simulink model "CrazyClover_attitude_control_descrete"  (R2020b)
settings: Solver=FixedStepDiscrete  StartTime=0.0  StopTime=1  FixedStep=0.01  RelTol=1e-3
values from neighbouring files (symbols this model uses):
  controller_matrix = [mass/(4*gravity)*1000 mass/(4*gravity)*1000 mass/(4*gravity)*1000 mass/(4*gravity)*1000 ... (first row only)    [sim_param.m]
  kM1 = Armlength /sqrt(2)    [sim_param.m]
  kM2 = Armlength /sqrt(2)    [sim_param.m]
  kM3 = 1    [sim_param.m]
undefined symbols (not defined in the file or in its folder): DiscIntNeverNeededParam, Pitch, Pitchrate, Roll, Rollrate, Yaw, Yawrate
libraries: pid_lib x18
(part 1 of 2)
settings Model: Creator=kt012  LastModifiedBy=kt012

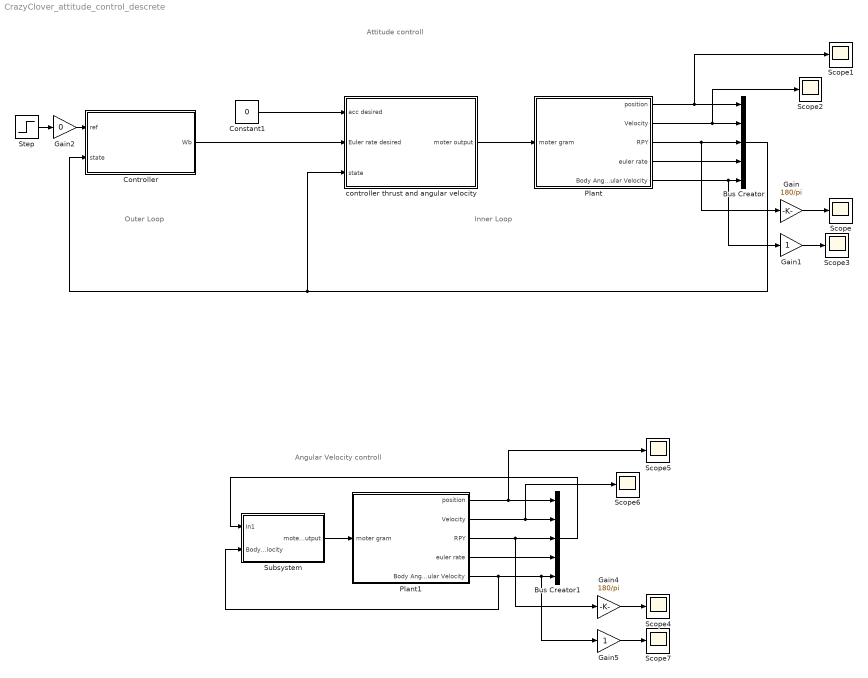
== system CrazyClover_attitude_control_descrete ==
  note: Inner Loop
  note: Outer Loop
  note: Attitude controll
  note: Angular Velocity controll
  Bus Creator : BusCreator  Inputs=5
  Bus Creator1 : BusCreator  Inputs=5
  Constant1 : Constant  Value=0
  Controller : Subsystem
  Gain : Gain  Gain=180/pi
  Gain1 : Gain
  Gain2 : Gain  Gain=0
  Gain4 : Gain  Gain=180/pi
  Gain5 : Gain
  Plant : Subsystem
  Plant1 : Subsystem
  Scope{,1..7} (8 alike) : Scope
  Step : Step  Time=5  Before=[0 0 0]'  After=[1 0 0]'  SampleTime=0
  Subsystem : Subsystem
  controller thrust and angular velocity : Subsystem
  wires:
  Controller/1(Wb) -> controller thrust and angular velocity/2(Euler rate desired)
  Constant1/1 -> controller thrust and angular velocity/1(acc desired)
  Step/1 -> Gain2/1
  Plant/4(euler rate) -> Bus Creator/4
  Plant/2(Velocity) -> Bus Creator/2, Scope2/1
  Plant/3(RPY) -> Gain/1, Bus Creator/3
  Plant/1(position) -> Bus Creator/1, Scope1/1
  controller thrust and angular velocity/1(moter output) -> Plant/1(moter gram)
  Bus Creator/1 -> controller thrust and angular velocity/3(state), Controller/2(state)
  Plant/5(Body Angular Velocity) -> Gain1/1, Bus Creator/5
  Gain/1 -> Scope/1
  Gain1/1 -> Scope3/1
  Gain2/1 -> Controller/1(ref)
  Gain4/1 -> Scope4/1
  Plant1/3(RPY) -> Gain4/1, Bus Creator1/3
  Plant1/5(Body Angular Velocity) -> Subsystem/2(Body Angular Velocity), Gain5/1, Bus Creator1/5
  Plant1/2(Velocity) -> Bus Creator1/2, Scope6/1
  Bus Creator1/1 -> Subsystem/1(In1)
  Plant1/1(position) -> Bus Creator1/1, Scope5/1
  Gain5/1 -> Scope7/1
  Plant1/4(euler rate) -> Bus Creator1/4
  Subsystem/1(moter output) -> Plant1/1(moter gram)

== system CrazyClover_attitude_control_descrete/Controller ==
  ref : Inport
  state : Inport  Port=2
  Subsystem3 : Subsystem
  Wb : Outport
  wires:
  ref/1 -> Subsystem3/1(RPY ref)
  Subsystem3/1(Wb) -> Wb/1
  state/1 -> Subsystem3/2(state)

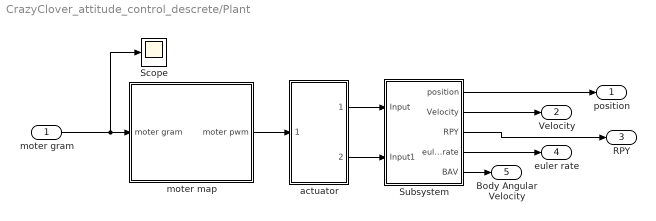
== system CrazyClover_attitude_control_descrete/Plant ==
  moter gram : Inport
  Scope : Scope
  Subsystem : Subsystem
  actuator : Subsystem
  moter map : Subsystem
  position : Outport
  Velocity : Outport  Port=2
  RPY : Outport  Port=3
  euler rate : Outport  Port=4
  Body Angular Velocity : Outport  Port=5
  wires:
  Subsystem/5(BAV) -> Body Angular Velocity/1
  Subsystem/1(position) -> position/1
  Subsystem/3(RPY) -> RPY/1
  moter gram/1 -> Scope/1, moter map/1(moter gram)
  actuator/2(Input1) -> Subsystem/2(Input1)
  actuator/1(Input) -> Subsystem/1(Input)
  moter map/1(moter pwm) -> actuator/1(PWM)
  Subsystem/4(euler rate) -> euler rate/1
  Subsystem/2(Velocity) -> Velocity/1

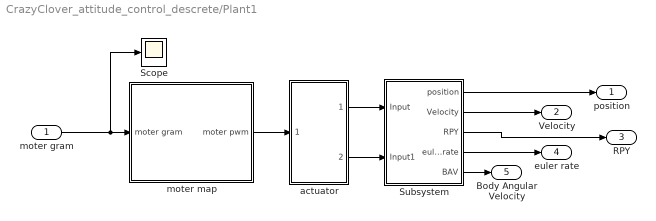
== system CrazyClover_attitude_control_descrete/Plant1 ==
  moter gram : Inport
  Scope : Scope
  Subsystem : Subsystem
  actuator : Subsystem
  moter map : Subsystem
  position : Outport
  Velocity : Outport  Port=2
  RPY : Outport  Port=3
  euler rate : Outport  Port=4
  Body Angular Velocity : Outport  Port=5
  wires:
  moter gram/1 -> Scope/1, moter map/1(moter gram)
  actuator/2(Input1) -> Subsystem/2(Input1)
  Subsystem/4(euler rate) -> euler rate/1
  moter map/1(moter pwm) -> actuator/1(PWM)
  Subsystem/2(Velocity) -> Velocity/1
  Subsystem/3(RPY) -> RPY/1
  Subsystem/1(position) -> position/1
  actuator/1(Input) -> Subsystem/1(Input)
  Subsystem/5(BAV) -> Body Angular Velocity/1

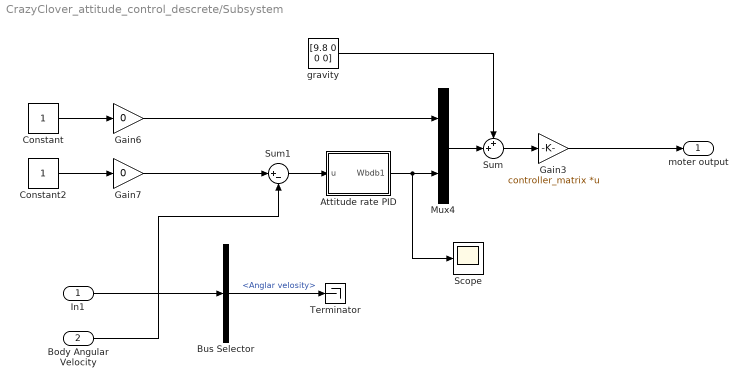
== system CrazyClover_attitude_control_descrete/Subsystem ==
  In1 : Inport
  Body Angular Velocity : Inport  Port=2
  Attitude rate PID : Subsystem
  Bus Selector : BusSelector  OutputSignals=Anglar velosity
  Constant : Constant
  Constant2 : Constant
  Gain3 : Gain  Gain=controller_matrix  Multiplication=Matrix(K*u)
  Gain6 : Gain  Gain=0
  Gain7 : Gain  Gain=0
  Mux4 : Mux  Inputs=2
  Scope : Scope
  Sum : Sum  Inputs=++|
  Sum1 : Sum  Inputs=|+-
  Terminator : Terminator
  gravity : Constant  Value=[9.8 0 0 0]
  moter output : Outport
  wires:
  Attitude rate PID/1(Wbdb1) -> Scope/1, Mux4/2
  Sum/1 -> Gain3/1
  Gain6/1 -> Mux4/1
  Mux4/1 -> Sum/2
  gravity/1 -> Sum/1
  Sum1/1 -> Attitude rate PID/1(u)
  Gain3/1 -> moter output/1
  Constant/1 -> Gain6/1
  Constant2/1 -> Gain7/1
  Gain7/1 -> Sum1/1
  In1/1 -> Bus Selector/1
  Bus Selector/1 -> Terminator/1  "<Anglar velosity>"
  Body Angular Velocity/1 -> Sum1/2

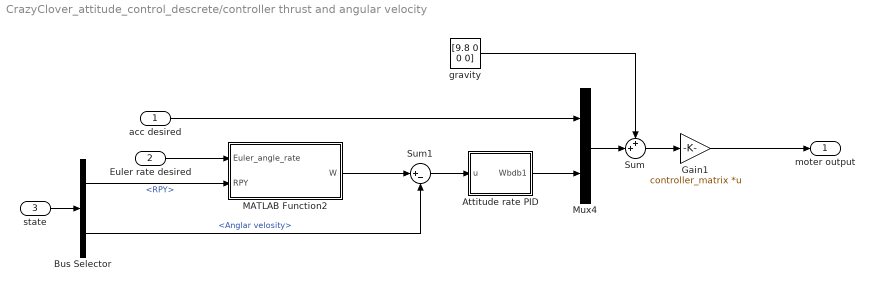
== system CrazyClover_attitude_control_descrete/controller thrust and angular velocity ==
  acc desired : Inport
  Euler rate desired : Inport  Port=2
  state : Inport  Port=3
  Attitude rate PID : Subsystem
  Bus Selector : BusSelector  OutputSignals=RPY,Anglar velosity
  Gain1 : Gain  Gain=controller_matrix  Multiplication=Matrix(K*u)
  MATLAB Function2 : MATLAB Function  TreatAsAtomicUnit=on
  Mux4 : Mux  Inputs=2
  Sum : Sum  Inputs=++|
  Sum1 : Sum  Inputs=|+-
  gravity : Constant  Value=[9.8 0 0 0]
  moter output : Outport
  wires:
  Sum/1 -> Gain1/1
  Gain1/1 -> moter output/1
  Mux4/1 -> Sum/2
  gravity/1 -> Sum/1
  Attitude rate PID/1(Wbdb1) -> Mux4/2
  state/1 -> Bus Selector/1
  Bus Selector/2 -> Sum1/2  "<Anglar velosity>"
  Sum1/1 -> Attitude rate PID/1(u)
  Euler rate desired/1 -> MATLAB Function2/1(Euler_angle_rate)
  acc desired/1 -> Mux4/1
  Bus Selector/1 -> MATLAB Function2/2(RPY)  "<RPY>"
  MATLAB Function2/1(W) -> Sum1/1

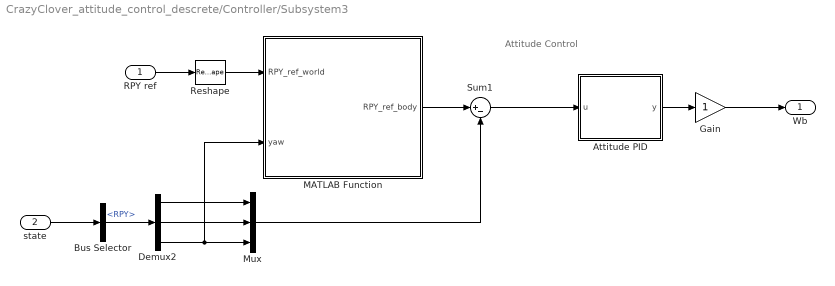
== system CrazyClover_attitude_control_descrete/Controller/Subsystem3 ==
  note: Attitude Control
  RPY ref : Inport
  state : Inport  Port=2
  Attitude PID : Subsystem
  Bus Selector : BusSelector  OutputSignals=RPY
  Demux2 : Demux  Outputs=3
  Gain : Gain
  MATLAB Function : MATLAB Function  TreatAsAtomicUnit=on
  Mux : Mux  Inputs=3
  Reshape : Reshape  OutputDimensionality=Row vector (2-D)
  Sum1 : Sum  Inputs=|+-
  Wb : Outport
  wires:
  Attitude PID/1(y) -> Gain/1
  MATLAB Function/1(RPY_ref_body) -> Sum1/1
  Sum1/1 -> Attitude PID/1(u)
  RPY ref/1 -> Reshape/1
  Demux2/3 -> MATLAB Function/2(yaw), Mux/3
  state/1 -> Bus Selector/1
  Bus Selector/1 -> Demux2/1  "<RPY>"
  Demux2/1 -> Mux/1
  Mux/1 -> Sum1/2
  Demux2/2 -> Mux/2
  Reshape/1 -> MATLAB Function/1(RPY_ref_world)
  Gain/1 -> Wb/1

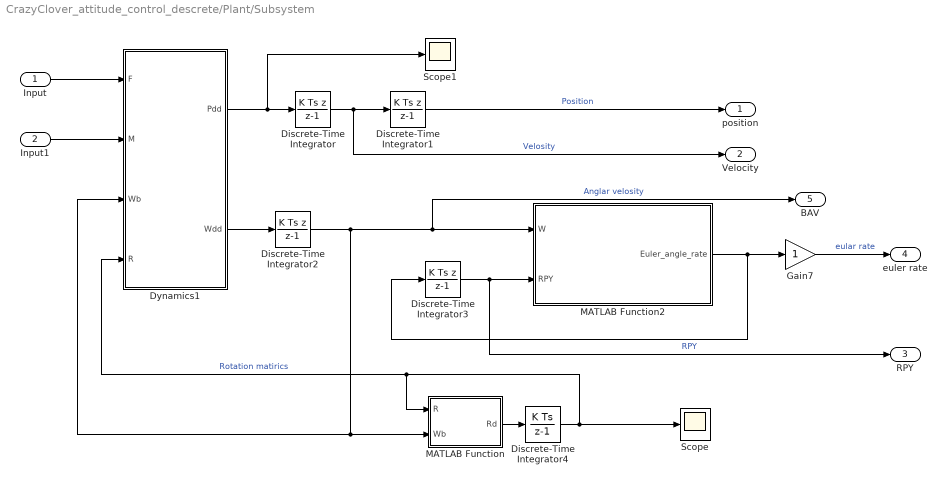
== system CrazyClover_attitude_control_descrete/Plant/Subsystem ==
  Input : Inport
  Input1 : Inport  Port=2
  Discrete-Time Integrator : DiscreteIntegrator  IntegratorMethod=Integration: Backward Euler  InitialCondition=[0 0 0]  SampleTime=-1  ICPrevOutput=DiscIntNeverNeededParam  ICPrevScaledInput=DiscIntNeverNeededParam
  Discrete-Time Integrator1 : DiscreteIntegrator  IntegratorMethod=Integration: Backward Euler  InitialCondition=[0 0 0]  SampleTime=-1  ICPrevOutput=DiscIntNeverNeededParam  ICPrevScaledInput=DiscIntNeverNeededParam
  Discrete-Time Integrator2 : DiscreteIntegrator  IntegratorMethod=Integration: Backward Euler  InitialCondition=[0 0 0]  SampleTime=-1  ICPrevOutput=DiscIntNeverNeededParam  ICPrevScaledInput=DiscIntNeverNeededParam
  Discrete-Time Integrator3 : DiscreteIntegrator  IntegratorMethod=Integration: Backward Euler  InitialCondition=[1 0 0]  SampleTime=-1  ICPrevOutput=DiscIntNeverNeededParam  ICPrevScaledInput=DiscIntNeverNeededParam
  Discrete-Time Integrator4 : DiscreteIntegrator  InitialCondition=[1 0 0; 0 1 0; 0 0 1]  SampleTime=-1  ICPrevOutput=DiscIntNeverNeededParam  ICPrevScaledInput=DiscIntNeverNeededParam
  Dynamics1 : MATLAB Function  TreatAsAtomicUnit=on
  Gain7 : Gain
  MATLAB Function : MATLAB Function  TreatAsAtomicUnit=on
  MATLAB Function2 : MATLAB Function  TreatAsAtomicUnit=on
  Scope : Scope
  Scope1 : Scope
  position : Outport
  Velocity : Outport  Port=2
  RPY : Outport  Port=3
  euler rate : Outport  Port=4
  BAV : Outport  Port=5
  wires:
  MATLAB Function2/1(Euler_angle_rate) -> Discrete-Time Integrator3/1, Gain7/1
  Dynamics1/1(Pdd) -> Discrete-Time Integrator/1, Scope1/1
  Discrete-Time Integrator1/1 -> position/1  "Position"
  Discrete-Time Integrator/1 -> Discrete-Time Integrator1/1, Velocity/1  "Velosity"
  Discrete-Time Integrator3/1 -> RPY/1, MATLAB Function2/2(RPY)  "RPY"
  Dynamics1/2(Wdd) -> Discrete-Time Integrator2/1
  Gain7/1 -> euler rate/1  "eular rate"
  MATLAB Function/1(Rd) -> Discrete-Time Integrator4/1
  Discrete-Time Integrator2/1 -> BAV/1, MATLAB Function2/1(W), MATLAB Function/2(Wb), Dynamics1/3(Wb)  "Anglar velosity"
  Discrete-Time Integrator4/1 -> Dynamics1/4(R), MATLAB Function/1(R), Scope/1  "Rotation matirics"
  Input1/1 -> Dynamics1/2(M)
  Input/1 -> Dynamics1/1(F)

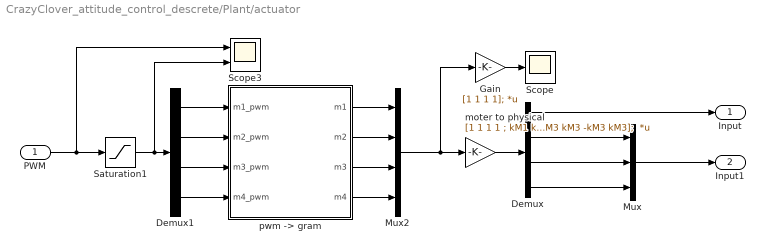
== system CrazyClover_attitude_control_descrete/Plant/actuator ==
  PWM : Inport
  Demux : Demux
  Demux1 : Demux
  Gain : Gain  Gain=[1 1 1 1];  Multiplication=Matrix(K*u)
  Mux : Mux  Inputs=3
  Mux2 : Mux
  Saturation1 : Saturate  UpperLimit=40000  LowerLimit=0
  Scope : Scope
  Scope3 : Scope  NumInputPorts=2
  moter to physical : Gain  Gain=[1 1 1 1 ; kM1 kM1 -kM1 -kM1; -kM2 kM2 kM2 -kM2; -kM3 kM3 -kM3 kM3];  Multiplication=Matrix(K*u)
  "pwm -> gram" : MATLAB Function  TreatAsAtomicUnit=on
  Input : Outport
  Input1 : Outport  Port=2
  wires:
  Demux/2 -> Mux/1
  "pwm -> gram"/3(m3) -> Mux2/3
  Demux1/2 -> "pwm -> gram"/2(m2_pwm)
  Demux/4 -> Mux/3
  Demux/3 -> Mux/2
  moter to physical/1 -> Demux/1
  "pwm -> gram"/1(m1) -> Mux2/1
  Mux2/1 -> Gain/1, moter to physical/1
  Gain/1 -> Scope/1
  Saturation1/1 -> Scope3/2, Demux1/1
  PWM/1 -> Scope3/1, Saturation1/1
  Demux1/3 -> "pwm -> gram"/3(m3_pwm)
  "pwm -> gram"/4(m4) -> Mux2/4
  "pwm -> gram"/2(m2) -> Mux2/2
  Demux1/4 -> "pwm -> gram"/4(m4_pwm)
  Demux1/1 -> "pwm -> gram"/1(m1_pwm)
  Mux/1 -> Input1/1
  Demux/1 -> Input/1

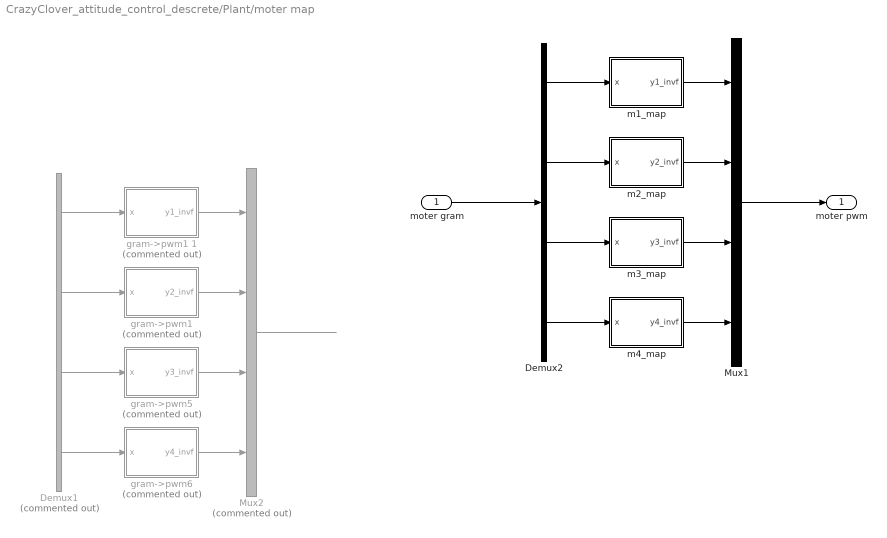
== system CrazyClover_attitude_control_descrete/Plant/moter map ==
  moter gram : Inport
  Demux1 : Demux  Commented=on
  Demux2 : Demux
  Mux1 : Mux
  Mux2 : Mux  Commented=on
  gram->pwm1 : MATLAB Function  Commented=on  TreatAsAtomicUnit=on
  gram->pwm1 1 : MATLAB Function  Commented=on  TreatAsAtomicUnit=on
  gram->pwm5 : MATLAB Function  Commented=on  TreatAsAtomicUnit=on
  gram->pwm6 : MATLAB Function  Commented=on  TreatAsAtomicUnit=on
  m1_map : MATLAB Function  TreatAsAtomicUnit=on
  m2_map : MATLAB Function  TreatAsAtomicUnit=on
  m3_map : MATLAB Function  TreatAsAtomicUnit=on
  m4_map : MATLAB Function  TreatAsAtomicUnit=on
  moter pwm : Outport
  wires:
  Demux2/4 -> m4_map/1(x)
  Demux2/3 -> m3_map/1(x)
  m4_map/1(y4_invf) -> Mux1/4
  Demux2/2 -> m2_map/1(x)
  m3_map/1(y3_invf) -> Mux1/3
  m2_map/1(y2_invf) -> Mux1/2
  m1_map/1(y1_invf) -> Mux1/1
  Demux2/1 -> m1_map/1(x)
  Mux1/1 -> moter pwm/1
  moter gram/1 -> Demux2/1
  ? -> Demux1/1
  Mux2/1 -> ?
  Demux1/1 -> gram->pwm1 1/1(x)
  gram->pwm1 1/1(y1_invf) -> Mux2/1
  gram->pwm1/1(y2_invf) -> Mux2/2
  gram->pwm5/1(y3_invf) -> Mux2/3
  Demux1/2 -> gram->pwm1/1(x)
  gram->pwm6/1(y4_invf) -> Mux2/4
  Demux1/3 -> gram->pwm5/1(x)
  Demux1/4 -> gram->pwm6/1(x)

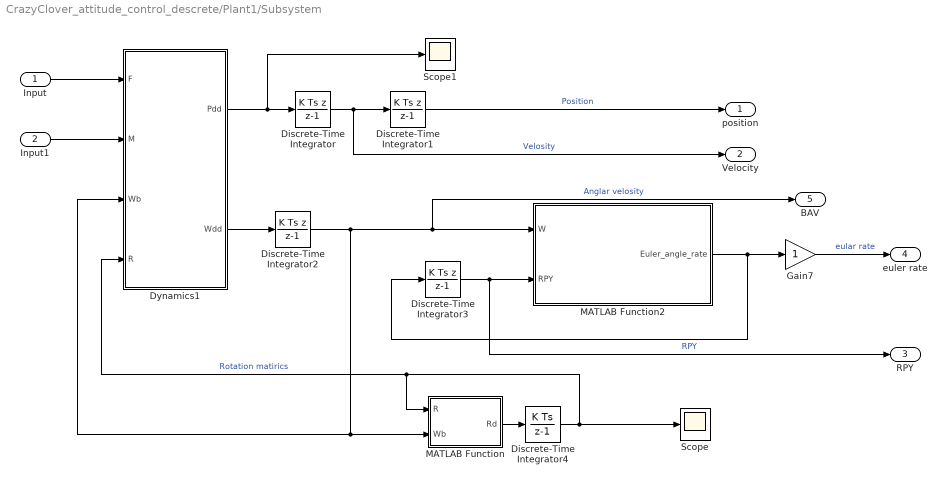
== system CrazyClover_attitude_control_descrete/Plant1/Subsystem ==
  Input : Inport
  Input1 : Inport  Port=2
  Discrete-Time Integrator : DiscreteIntegrator  IntegratorMethod=Integration: Backward Euler  InitialCondition=[0 0 0]  SampleTime=-1  ICPrevOutput=DiscIntNeverNeededParam  ICPrevScaledInput=DiscIntNeverNeededParam
  Discrete-Time Integrator1 : DiscreteIntegrator  IntegratorMethod=Integration: Backward Euler  InitialCondition=[0 0 0]  SampleTime=-1  ICPrevOutput=DiscIntNeverNeededParam  ICPrevScaledInput=DiscIntNeverNeededParam
  Discrete-Time Integrator2 : DiscreteIntegrator  IntegratorMethod=Integration: Backward Euler  InitialCondition=[1 0 0]  SampleTime=-1  ICPrevOutput=DiscIntNeverNeededParam  ICPrevScaledInput=DiscIntNeverNeededParam
  Discrete-Time Integrator3 : DiscreteIntegrator  IntegratorMethod=Integration: Backward Euler  InitialCondition=[0 0 0]  SampleTime=-1  ICPrevOutput=DiscIntNeverNeededParam  ICPrevScaledInput=DiscIntNeverNeededParam
  Discrete-Time Integrator4 : DiscreteIntegrator  InitialCondition=[1 0 0; 0 1 0; 0 0 1]  SampleTime=-1  ICPrevOutput=DiscIntNeverNeededParam  ICPrevScaledInput=DiscIntNeverNeededParam
  Dynamics1 : MATLAB Function  TreatAsAtomicUnit=on
  Gain7 : Gain
  MATLAB Function : MATLAB Function  TreatAsAtomicUnit=on
  MATLAB Function2 : MATLAB Function  TreatAsAtomicUnit=on
  Scope : Scope
  Scope1 : Scope
  position : Outport
  Velocity : Outport  Port=2
  RPY : Outport  Port=3
  euler rate : Outport  Port=4
  BAV : Outport  Port=5
  wires:
  MATLAB Function2/1(Euler_angle_rate) -> Discrete-Time Integrator3/1, Gain7/1
  Dynamics1/1(Pdd) -> Discrete-Time Integrator/1, Scope1/1
  Discrete-Time Integrator1/1 -> position/1  "Position"
  Discrete-Time Integrator/1 -> Discrete-Time Integrator1/1, Velocity/1  "Velosity"
  Discrete-Time Integrator3/1 -> RPY/1, MATLAB Function2/2(RPY)  "RPY"
  Dynamics1/2(Wdd) -> Discrete-Time Integrator2/1
  Gain7/1 -> euler rate/1  "eular rate"
  MATLAB Function/1(Rd) -> Discrete-Time Integrator4/1
  Discrete-Time Integrator2/1 -> BAV/1, MATLAB Function2/1(W), MATLAB Function/2(Wb), Dynamics1/3(Wb)  "Anglar velosity"
  Discrete-Time Integrator4/1 -> Dynamics1/4(R), MATLAB Function/1(R), Scope/1  "Rotation matirics"
  Input1/1 -> Dynamics1/2(M)
  Input/1 -> Dynamics1/1(F)

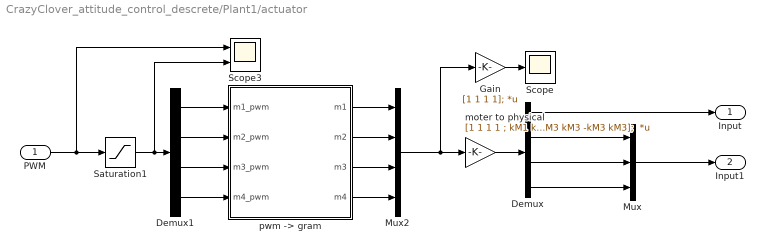
== system CrazyClover_attitude_control_descrete/Plant1/actuator ==
  PWM : Inport
  Demux : Demux
  Demux1 : Demux
  Gain : Gain  Gain=[1 1 1 1];  Multiplication=Matrix(K*u)
  Mux : Mux  Inputs=3
  Mux2 : Mux
  Saturation1 : Saturate  UpperLimit=40000  LowerLimit=0
  Scope : Scope
  Scope3 : Scope  NumInputPorts=2
  moter to physical : Gain  Gain=[1 1 1 1 ; kM1 kM1 -kM1 -kM1; -kM2 kM2 kM2 -kM2; -kM3 kM3 -kM3 kM3];  Multiplication=Matrix(K*u)
  "pwm -> gram" : MATLAB Function  TreatAsAtomicUnit=on
  Input : Outport
  Input1 : Outport  Port=2
  wires:
  Demux/2 -> Mux/1
  "pwm -> gram"/3(m3) -> Mux2/3
  Demux1/2 -> "pwm -> gram"/2(m2_pwm)
  Demux/4 -> Mux/3
  Demux/3 -> Mux/2
  moter to physical/1 -> Demux/1
  "pwm -> gram"/1(m1) -> Mux2/1
  Mux2/1 -> Gain/1, moter to physical/1
  Gain/1 -> Scope/1
  Saturation1/1 -> Scope3/2, Demux1/1
  PWM/1 -> Scope3/1, Saturation1/1
  Demux1/3 -> "pwm -> gram"/3(m3_pwm)
  "pwm -> gram"/4(m4) -> Mux2/4
  "pwm -> gram"/2(m2) -> Mux2/2
  Demux1/4 -> "pwm -> gram"/4(m4_pwm)
  Demux1/1 -> "pwm -> gram"/1(m1_pwm)
  Mux/1 -> Input1/1
  Demux/1 -> Input/1

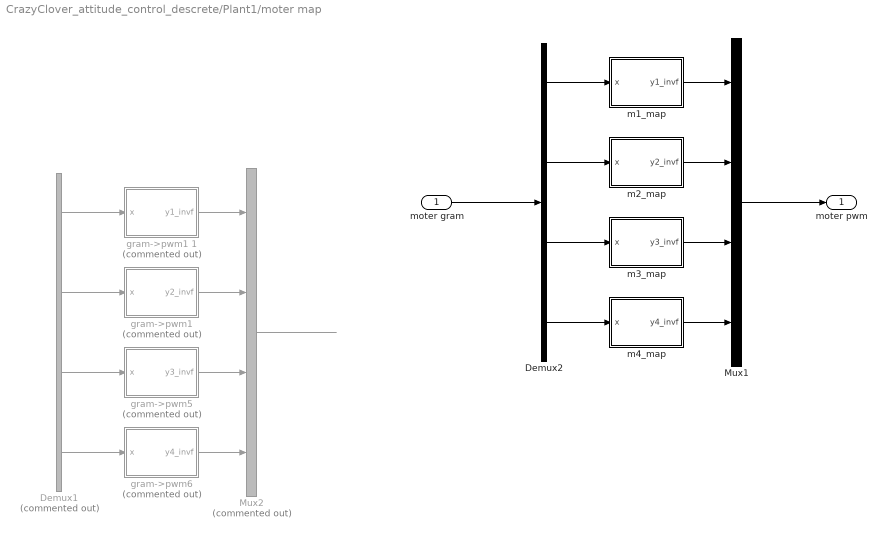
== system CrazyClover_attitude_control_descrete/Plant1/moter map ==
  moter gram : Inport
  Demux1 : Demux  Commented=on
  Demux2 : Demux
  Mux1 : Mux
  Mux2 : Mux  Commented=on
  gram->pwm1 : MATLAB Function  Commented=on  TreatAsAtomicUnit=on
  gram->pwm1 1 : MATLAB Function  Commented=on  TreatAsAtomicUnit=on
  gram->pwm5 : MATLAB Function  Commented=on  TreatAsAtomicUnit=on
  gram->pwm6 : MATLAB Function  Commented=on  TreatAsAtomicUnit=on
  m1_map : MATLAB Function  TreatAsAtomicUnit=on
  m2_map : MATLAB Function  TreatAsAtomicUnit=on
  m3_map : MATLAB Function  TreatAsAtomicUnit=on
  m4_map : MATLAB Function  TreatAsAtomicUnit=on
  moter pwm : Outport
  wires:
  Demux2/4 -> m4_map/1(x)
  Demux2/3 -> m3_map/1(x)
  m4_map/1(y4_invf) -> Mux1/4
  Demux2/2 -> m2_map/1(x)
  m3_map/1(y3_invf) -> Mux1/3
  m2_map/1(y2_invf) -> Mux1/2
  m1_map/1(y1_invf) -> Mux1/1
  Demux2/1 -> m1_map/1(x)
  Mux1/1 -> moter pwm/1
  moter gram/1 -> Demux2/1
  ? -> Demux1/1
  Mux2/1 -> ?
  Demux1/1 -> gram->pwm1 1/1(x)
  gram->pwm1 1/1(y1_invf) -> Mux2/1
  gram->pwm1/1(y2_invf) -> Mux2/2
  gram->pwm5/1(y3_invf) -> Mux2/3
  Demux1/2 -> gram->pwm1/1(x)
  gram->pwm6/1(y4_invf) -> Mux2/4
  Demux1/3 -> gram->pwm5/1(x)
  Demux1/4 -> gram->pwm6/1(x)

== system CrazyClover_attitude_control_descrete/Subsystem/Attitude rate PID ==
  u : Inport
  Demux : Demux  Outputs=3
  Mux1 : Mux  Inputs=3
  "Yaw rate PID " : Subsystem
  pitch rate PID : Subsystem
  "roll rate PID " : Subsystem
  Wbdb1 : Outport
  wires:
  "roll rate PID "/1(y) -> Mux1/1
  pitch rate PID/1(y) -> Mux1/2
  Demux/2 -> pitch rate PID/1(u)
  u/1 -> Demux/1
  Demux/3 -> "Yaw rate PID "/1(u)
  Demux/1 -> "roll rate PID "/1(u)
  "Yaw rate PID "/1(y) -> Mux1/3
  Mux1/1 -> Wbdb1/1

== system CrazyClover_attitude_control_descrete/controller thrust and angular velocity/Attitude rate PID ==
  u : Inport
  Demux : Demux  Outputs=3
  Mux1 : Mux  Inputs=3
  "Yaw rate PID " : Subsystem
  pitch rate PID : Subsystem
  "roll rate PID " : Subsystem
  Wbdb1 : Outport
  wires:
  "roll rate PID "/1(y) -> Mux1/1
  pitch rate PID/1(y) -> Mux1/2
  Demux/2 -> pitch rate PID/1(u)
  u/1 -> Demux/1
  Demux/3 -> "Yaw rate PID "/1(u)
  Demux/1 -> "roll rate PID "/1(u)
  "Yaw rate PID "/1(y) -> Mux1/3
  Mux1/1 -> Wbdb1/1

== system CrazyClover_attitude_control_descrete/Controller/Subsystem3/Attitude PID ==
  u : Inport
  Demux1 : Demux  Outputs=3
  Mux2 : Mux  Inputs=3
  "Yaw PID " : Subsystem
  pitch PID : Subsystem
  roll PID : Subsystem
  y : Outport
  wires:
  roll PID/1(y) -> Mux2/1
  pitch PID/1(y) -> Mux2/2
  Mux2/1 -> y/1
  u/1 -> Demux1/1  "Euler angle"
  Demux1/2 -> pitch PID/1(u)
  Demux1/1 -> roll PID/1(u)
  "Yaw PID "/1(y) -> Mux2/3
  Demux1/3 -> "Yaw PID "/1(u)

== system CrazyClover_attitude_control_descrete/Subsystem/Attitude rate PID/Yaw rate PID  ==
  u : Inport
  PID Controller : pid_lib/PID Controller  Controller=PID  Form=Parallel  TimeDomain=Discrete-time  UseExternalTs=off  SampleTime=-1  IntegratorMethod=Forward Euler  FilterMethod=Forward Euler  ControllerParametersSource=internal  P=0  I=Yawrate.ki  D=0  UseFilter=on  N=100  TunerSelectOption=Transfer Function Based (PID Tuner App)  InitialConditionSource=internal  InitialConditionForIntegrator=0  InitialConditionForFilter=0  DifferentiatorICPrevScaledInput=0  ExternalReset=none  TrackingMode=off  Kt=1  LimitOutput=off  SatLimitsSource=internal  UpperSaturationLimit=inf  LowerSaturationLimit=-inf  LinearizeAsGain=on  AntiWindupMode=none  Kb=1  POutMin=[]  POutMax=[]  IOutMin=[]  IOutMax=[]  DOutMin=[]  DOutMax=[]  NOutMin=[]  NOutMax=[]  SumOutMin=[]  SumOutMax=[]  SaturationOutMin=[]  SaturationOutMax=[]  PParamMin=[]  PParamMax=[]  IParamMin=[]  IParamMax=[]  DParamMin=[]  DParamMax=[]  NParamMin=[]  NParamMax=[]  KbParamMin=[]  KbParamMax=[]  KtParamMin=[]  KtParamMax=[]  KbOutMin=[]  KbOutMax=[]  KtOutMin=[]  KtOutMax=[]  IntegratorOutMin=[]  IntegratorOutMax=[]  FilterOutMin=[]  FilterOutMax=[]  SumI1OutMin=[]  SumI1OutMax=[]  SumI2OutMin=[]  SumI2OutMax=[]  SumI3OutMin=[]  SumI3OutMax=[]  SumI4OutMin=[]  SumI4OutMax=[]  SumDOutMin=[]  SumDOutMax=[]  DifferentiatorOutMin=[]  DifferentiatorOutMax=[]  FilterDiffOutCoefMin=[]  FilterDiffOutCoefMax=[]  ReciprocalOutMin=[]  ReciprocalOutMax=[]  SumDenOutMin=[]  SumDenOutMax=[]  SumNumOutMin=[]  SumNumOutMax=[]  DivideOutMin=[]  DivideOutMax=[]  UdiffTsProdOutMin=[]  UdiffTsProdOutMax=[]  NTsProdOutMin=[]  NTsProdOutMax=[]  UintegralTsProdOutMin=[]  UintegralTsProdOutMax=[]  UngainTsProdOutMin=[]  UngainTsProdOutMax=[]  IntegratorContinuousStateAttributes=''  IntegratorStateMustResolveToSignalObject=off  IntegratorRTWStateStorageClass=Auto  FilterContinuousStateAttributes=''  FilterStateMustResolveToSignalObject=off  FilterRTWStateStorageClass=Auto  ParallelPVariant=InternalParameters  IdealPVariant=Disabled  IVariant=InternalParameters  DVariant=InternalParameters  IntegratorVariant=Discrete  SatVariant=Disabled  AWVariant=Passthrough  PCopyVariant=Disabled  TRVariant=Disabled  FdbkBlocksVariant=Forward  IdealPFdbkVariant=Disabled  SatFdbkVariant=Disabled  DerivativeFilterVariant=ForwardEulerFilter  NVariant=InternalParameters  NCopyVariant=Disabled  FilterICVariant=InternalICsFilter  IntegratorICVariant=InternalICs  ExternalResetVariant=Disabled  TRSumVariant=Passthrough  SumFdbkVariant=Disabled  SumVariant=Sum_PID  TsampFilterVariant=InternalTs  TsampNgainVariant=Passthrough  TsampIntegralVariant=Passthrough  ExternalSaturationOutDataTypeStr=Inherit: Same as second input
  PID Controller2 : pid_lib/PID Controller  Controller=PID  Form=Parallel  TimeDomain=Discrete-time  UseExternalTs=off  SampleTime=-1  IntegratorMethod=Forward Euler  FilterMethod=Forward Euler  ControllerParametersSource=internal  P=Yawrate.kp  I=0  D=0  UseFilter=on  N=100  TunerSelectOption=Transfer Function Based (PID Tuner App)  InitialConditionSource=internal  InitialConditionForIntegrator=0  InitialConditionForFilter=0  DifferentiatorICPrevScaledInput=0  ExternalReset=none  TrackingMode=off  Kt=1  LimitOutput=off  SatLimitsSource=internal  UpperSaturationLimit=inf  LowerSaturationLimit=-inf  LinearizeAsGain=on  AntiWindupMode=none  Kb=1  POutMin=[]  POutMax=[]  IOutMin=[]  IOutMax=[]  DOutMin=[]  DOutMax=[]  NOutMin=[]  NOutMax=[]  SumOutMin=[]  SumOutMax=[]  SaturationOutMin=[]  SaturationOutMax=[]  PParamMin=[]  PParamMax=[]  IParamMin=[]  IParamMax=[]  DParamMin=[]  DParamMax=[]  NParamMin=[]  NParamMax=[]  KbParamMin=[]  KbParamMax=[]  KtParamMin=[]  KtParamMax=[]  KbOutMin=[]  KbOutMax=[]  KtOutMin=[]  KtOutMax=[]  IntegratorOutMin=[]  IntegratorOutMax=[]  FilterOutMin=[]  FilterOutMax=[]  SumI1OutMin=[]  SumI1OutMax=[]  SumI2OutMin=[]  SumI2OutMax=[]  SumI3OutMin=[]  SumI3OutMax=[]  SumI4OutMin=[]  SumI4OutMax=[]  SumDOutMin=[]  SumDOutMax=[]  DifferentiatorOutMin=[]  DifferentiatorOutMax=[]  FilterDiffOutCoefMin=[]  FilterDiffOutCoefMax=[]  ReciprocalOutMin=[]  ReciprocalOutMax=[]  SumDenOutMin=[]  SumDenOutMax=[]  SumNumOutMin=[]  SumNumOutMax=[]  DivideOutMin=[]  DivideOutMax=[]  UdiffTsProdOutMin=[]  UdiffTsProdOutMax=[]  NTsProdOutMin=[]  NTsProdOutMax=[]  UintegralTsProdOutMin=[]  UintegralTsProdOutMax=[]  UngainTsProdOutMin=[]  UngainTsProdOutMax=[]  IntegratorContinuousStateAttributes=''  IntegratorStateMustResolveToSignalObject=off  IntegratorRTWStateStorageClass=Auto  FilterContinuousStateAttributes=''  FilterStateMustResolveToSignalObject=off  FilterRTWStateStorageClass=Auto  ParallelPVariant=InternalParameters  IdealPVariant=Disabled  IVariant=InternalParameters  DVariant=InternalParameters  IntegratorVariant=Discrete  SatVariant=Disabled  AWVariant=Passthrough  PCopyVariant=Disabled  TRVariant=Disabled  FdbkBlocksVariant=Forward  IdealPFdbkVariant=Disabled  SatFdbkVariant=Disabled  DerivativeFilterVariant=ForwardEulerFilter  NVariant=InternalParameters  NCopyVariant=Disabled  FilterICVariant=InternalICsFilter  IntegratorICVariant=InternalICs  ExternalResetVariant=Disabled  TRSumVariant=Passthrough  SumFdbkVariant=Disabled  SumVariant=Sum_PID  TsampFilterVariant=InternalTs  TsampNgainVariant=Passthrough  TsampIntegralVariant=Passthrough  ExternalSaturationOutDataTypeStr=Inherit: Same as second input
  Saturation : Saturate  UpperLimit=Yawrate.intupper  LowerLimit=Yawrate.intlower
  Scope : Scope  NumInputPorts=2
  Sum : Sum  Inputs=|++
  y : Outport
  wires:
  PID Controller2/1 -> Sum/1
  u/1 -> PID Controller/1, PID Controller2/1
  Sum/1 -> y/1
  PID Controller/1 -> Scope/2, Saturation/1
  Saturation/1 -> Sum/2, Scope/1

== system CrazyClover_attitude_control_descrete/Subsystem/Attitude rate PID/pitch rate PID ==
  u : Inport
  PID Controller1 : pid_lib/PID Controller  Controller=PID  Form=Parallel  TimeDomain=Discrete-time  UseExternalTs=off  SampleTime=-1  IntegratorMethod=Forward Euler  FilterMethod=Forward Euler  ControllerParametersSource=internal  P=0  I=Pitchrate.ki  D=0  UseFilter=on  N=100  TunerSelectOption=Transfer Function Based (PID Tuner App)  InitialConditionSource=internal  InitialConditionForIntegrator=0  InitialConditionForFilter=0  DifferentiatorICPrevScaledInput=0  ExternalReset=none  TrackingMode=off  Kt=1  LimitOutput=off  SatLimitsSource=internal  UpperSaturationLimit=inf  LowerSaturationLimit=-inf  LinearizeAsGain=on  AntiWindupMode=none  Kb=1  POutMin=[]  POutMax=[]  IOutMin=[]  IOutMax=[]  DOutMin=[]  DOutMax=[]  NOutMin=[]  NOutMax=[]  SumOutMin=[]  SumOutMax=[]  SaturationOutMin=[]  SaturationOutMax=[]  PParamMin=[]  PParamMax=[]  IParamMin=[]  IParamMax=[]  DParamMin=[]  DParamMax=[]  NParamMin=[]  NParamMax=[]  KbParamMin=[]  KbParamMax=[]  KtParamMin=[]  KtParamMax=[]  KbOutMin=[]  KbOutMax=[]  KtOutMin=[]  KtOutMax=[]  IntegratorOutMin=[]  IntegratorOutMax=[]  FilterOutMin=[]  FilterOutMax=[]  SumI1OutMin=[]  SumI1OutMax=[]  SumI2OutMin=[]  SumI2OutMax=[]  SumI3OutMin=[]  SumI3OutMax=[]  SumI4OutMin=[]  SumI4OutMax=[]  SumDOutMin=[]  SumDOutMax=[]  DifferentiatorOutMin=[]  DifferentiatorOutMax=[]  FilterDiffOutCoefMin=[]  FilterDiffOutCoefMax=[]  ReciprocalOutMin=[]  ReciprocalOutMax=[]  SumDenOutMin=[]  SumDenOutMax=[]  SumNumOutMin=[]  SumNumOutMax=[]  DivideOutMin=[]  DivideOutMax=[]  UdiffTsProdOutMin=[]  UdiffTsProdOutMax=[]  NTsProdOutMin=[]  NTsProdOutMax=[]  UintegralTsProdOutMin=[]  UintegralTsProdOutMax=[]  UngainTsProdOutMin=[]  UngainTsProdOutMax=[]  IntegratorContinuousStateAttributes=''  IntegratorStateMustResolveToSignalObject=off  IntegratorRTWStateStorageClass=Auto  FilterContinuousStateAttributes=''  FilterStateMustResolveToSignalObject=off  FilterRTWStateStorageClass=Auto  ParallelPVariant=InternalParameters  IdealPVariant=Disabled  IVariant=InternalParameters  DVariant=InternalParameters  IntegratorVariant=Discrete  SatVariant=Disabled  AWVariant=Passthrough  PCopyVariant=Disabled  TRVariant=Disabled  FdbkBlocksVariant=Forward  IdealPFdbkVariant=Disabled  SatFdbkVariant=Disabled  DerivativeFilterVariant=ForwardEulerFilter  NVariant=InternalParameters  NCopyVariant=Disabled  FilterICVariant=InternalICsFilter  IntegratorICVariant=InternalICs  ExternalResetVariant=Disabled  TRSumVariant=Passthrough  SumFdbkVariant=Disabled  SumVariant=Sum_PID  TsampFilterVariant=InternalTs  TsampNgainVariant=Passthrough  TsampIntegralVariant=Passthrough  ExternalSaturationOutDataTypeStr=Inherit: Same as second input
  PID Controller2 : pid_lib/PID Controller  Controller=PID  Form=Parallel  TimeDomain=Discrete-time  UseExternalTs=off  SampleTime=-1  IntegratorMethod=Forward Euler  FilterMethod=Forward Euler  ControllerParametersSource=internal  P=Pitchrate.kp  I=0  D=0  UseFilter=on  N=100  TunerSelectOption=Transfer Function Based (PID Tuner App)  InitialConditionSource=internal  InitialConditionForIntegrator=0  InitialConditionForFilter=0  DifferentiatorICPrevScaledInput=0  ExternalReset=none  TrackingMode=off  Kt=1  LimitOutput=off  SatLimitsSource=internal  UpperSaturationLimit=inf  LowerSaturationLimit=-inf  LinearizeAsGain=on  AntiWindupMode=none  Kb=1  POutMin=[]  POutMax=[]  IOutMin=[]  IOutMax=[]  DOutMin=[]  DOutMax=[]  NOutMin=[]  NOutMax=[]  SumOutMin=[]  SumOutMax=[]  SaturationOutMin=[]  SaturationOutMax=[]  PParamMin=[]  PParamMax=[]  IParamMin=[]  IParamMax=[]  DParamMin=[]  DParamMax=[]  NParamMin=[]  NParamMax=[]  KbParamMin=[]  KbParamMax=[]  KtParamMin=[]  KtParamMax=[]  KbOutMin=[]  KbOutMax=[]  KtOutMin=[]  KtOutMax=[]  IntegratorOutMin=[]  IntegratorOutMax=[]  FilterOutMin=[]  FilterOutMax=[]  SumI1OutMin=[]  SumI1OutMax=[]  SumI2OutMin=[]  SumI2OutMax=[]  SumI3OutMin=[]  SumI3OutMax=[]  SumI4OutMin=[]  SumI4OutMax=[]  SumDOutMin=[]  SumDOutMax=[]  DifferentiatorOutMin=[]  DifferentiatorOutMax=[]  FilterDiffOutCoefMin=[]  FilterDiffOutCoefMax=[]  ReciprocalOutMin=[]  ReciprocalOutMax=[]  SumDenOutMin=[]  SumDenOutMax=[]  SumNumOutMin=[]  SumNumOutMax=[]  DivideOutMin=[]  DivideOutMax=[]  UdiffTsProdOutMin=[]  UdiffTsProdOutMax=[]  NTsProdOutMin=[]  NTsProdOutMax=[]  UintegralTsProdOutMin=[]  UintegralTsProdOutMax=[]  UngainTsProdOutMin=[]  UngainTsProdOutMax=[]  IntegratorContinuousStateAttributes=''  IntegratorStateMustResolveToSignalObject=off  IntegratorRTWStateStorageClass=Auto  FilterContinuousStateAttributes=''  FilterStateMustResolveToSignalObject=off  FilterRTWStateStorageClass=Auto  ParallelPVariant=InternalParameters  IdealPVariant=Disabled  IVariant=InternalParameters  DVariant=InternalParameters  IntegratorVariant=Discrete  SatVariant=Disabled  AWVariant=Passthrough  PCopyVariant=Disabled  TRVariant=Disabled  FdbkBlocksVariant=Forward  IdealPFdbkVariant=Disabled  SatFdbkVariant=Disabled  DerivativeFilterVariant=ForwardEulerFilter  NVariant=InternalParameters  NCopyVariant=Disabled  FilterICVariant=InternalICsFilter  IntegratorICVariant=InternalICs  ExternalResetVariant=Disabled  TRSumVariant=Passthrough  SumFdbkVariant=Disabled  SumVariant=Sum_PID  TsampFilterVariant=InternalTs  TsampNgainVariant=Passthrough  TsampIntegralVariant=Passthrough  ExternalSaturationOutDataTypeStr=Inherit: Same as second input
  Saturation : Saturate  UpperLimit=Pitchrate.intupper  LowerLimit=Pitchrate.intlower
  Scope : Scope  NumInputPorts=2
  Sum : Sum  Inputs=|++
  y : Outport
  wires:
  PID Controller2/1 -> Sum/1
  u/1 -> PID Controller1/1, PID Controller2/1
  Sum/1 -> y/1
  PID Controller1/1 -> Scope/2, Saturation/1
  Saturation/1 -> Sum/2, Scope/1

== system CrazyClover_attitude_control_descrete/Subsystem/Attitude rate PID/roll rate PID  ==
  u : Inport
  PID Controller1 : pid_lib/PID Controller  Controller=PID  Form=Parallel  TimeDomain=Discrete-time  UseExternalTs=off  SampleTime=-1  IntegratorMethod=Forward Euler  FilterMethod=Forward Euler  ControllerParametersSource=internal  P=0  I=Rollrate.ki  D=0  UseFilter=on  N=100  TunerSelectOption=Transfer Function Based (PID Tuner App)  InitialConditionSource=internal  InitialConditionForIntegrator=0  InitialConditionForFilter=0  DifferentiatorICPrevScaledInput=0  ExternalReset=none  TrackingMode=off  Kt=1  LimitOutput=off  SatLimitsSource=internal  UpperSaturationLimit=inf  LowerSaturationLimit=-inf  LinearizeAsGain=on  AntiWindupMode=none  Kb=1  POutMin=[]  POutMax=[]  IOutMin=[]  IOutMax=[]  DOutMin=[]  DOutMax=[]  NOutMin=[]  NOutMax=[]  SumOutMin=[]  SumOutMax=[]  SaturationOutMin=[]  SaturationOutMax=[]  PParamMin=[]  PParamMax=[]  IParamMin=[]  IParamMax=[]  DParamMin=[]  DParamMax=[]  NParamMin=[]  NParamMax=[]  KbParamMin=[]  KbParamMax=[]  KtParamMin=[]  KtParamMax=[]  KbOutMin=[]  KbOutMax=[]  KtOutMin=[]  KtOutMax=[]  IntegratorOutMin=[]  IntegratorOutMax=[]  FilterOutMin=[]  FilterOutMax=[]  SumI1OutMin=[]  SumI1OutMax=[]  SumI2OutMin=[]  SumI2OutMax=[]  SumI3OutMin=[]  SumI3OutMax=[]  SumI4OutMin=[]  SumI4OutMax=[]  SumDOutMin=[]  SumDOutMax=[]  DifferentiatorOutMin=[]  DifferentiatorOutMax=[]  FilterDiffOutCoefMin=[]  FilterDiffOutCoefMax=[]  ReciprocalOutMin=[]  ReciprocalOutMax=[]  SumDenOutMin=[]  SumDenOutMax=[]  SumNumOutMin=[]  SumNumOutMax=[]  DivideOutMin=[]  DivideOutMax=[]  UdiffTsProdOutMin=[]  UdiffTsProdOutMax=[]  NTsProdOutMin=[]  NTsProdOutMax=[]  UintegralTsProdOutMin=[]  UintegralTsProdOutMax=[]  UngainTsProdOutMin=[]  UngainTsProdOutMax=[]  IntegratorContinuousStateAttributes=''  IntegratorStateMustResolveToSignalObject=off  IntegratorRTWStateStorageClass=Auto  FilterContinuousStateAttributes=''  FilterStateMustResolveToSignalObject=off  FilterRTWStateStorageClass=Auto  ParallelPVariant=InternalParameters  IdealPVariant=Disabled  IVariant=InternalParameters  DVariant=InternalParameters  IntegratorVariant=Discrete  SatVariant=Disabled  AWVariant=Passthrough  PCopyVariant=Disabled  TRVariant=Disabled  FdbkBlocksVariant=Forward  IdealPFdbkVariant=Disabled  SatFdbkVariant=Disabled  DerivativeFilterVariant=ForwardEulerFilter  NVariant=InternalParameters  NCopyVariant=Disabled  FilterICVariant=InternalICsFilter  IntegratorICVariant=InternalICs  ExternalResetVariant=Disabled  TRSumVariant=Passthrough  SumFdbkVariant=Disabled  SumVariant=Sum_PID  TsampFilterVariant=InternalTs  TsampNgainVariant=Passthrough  TsampIntegralVariant=Passthrough  ExternalSaturationOutDataTypeStr=Inherit: Same as second input
  PID Controller2 : pid_lib/PID Controller  Controller=PID  Form=Parallel  TimeDomain=Discrete-time  UseExternalTs=off  SampleTime=-1  IntegratorMethod=Forward Euler  FilterMethod=Forward Euler  ControllerParametersSource=internal  P=Rollrate.kp  I=0  D=0  UseFilter=on  N=100  TunerSelectOption=Transfer Function Based (PID Tuner App)  InitialConditionSource=internal  InitialConditionForIntegrator=0  InitialConditionForFilter=0  DifferentiatorICPrevScaledInput=0  ExternalReset=none  TrackingMode=off  Kt=1  LimitOutput=off  SatLimitsSource=internal  UpperSaturationLimit=inf  LowerSaturationLimit=-inf  LinearizeAsGain=on  AntiWindupMode=none  Kb=1  POutMin=[]  POutMax=[]  IOutMin=[]  IOutMax=[]  DOutMin=[]  DOutMax=[]  NOutMin=[]  NOutMax=[]  SumOutMin=[]  SumOutMax=[]  SaturationOutMin=[]  SaturationOutMax=[]  PParamMin=[]  PParamMax=[]  IParamMin=[]  IParamMax=[]  DParamMin=[]  DParamMax=[]  NParamMin=[]  NParamMax=[]  KbParamMin=[]  KbParamMax=[]  KtParamMin=[]  KtParamMax=[]  KbOutMin=[]  KbOutMax=[]  KtOutMin=[]  KtOutMax=[]  IntegratorOutMin=[]  IntegratorOutMax=[]  FilterOutMin=[]  FilterOutMax=[]  SumI1OutMin=[]  SumI1OutMax=[]  SumI2OutMin=[]  SumI2OutMax=[]  SumI3OutMin=[]  SumI3OutMax=[]  SumI4OutMin=[]  SumI4OutMax=[]  SumDOutMin=[]  SumDOutMax=[]  DifferentiatorOutMin=[]  DifferentiatorOutMax=[]  FilterDiffOutCoefMin=[]  FilterDiffOutCoefMax=[]  ReciprocalOutMin=[]  ReciprocalOutMax=[]  SumDenOutMin=[]  SumDenOutMax=[]  SumNumOutMin=[]  SumNumOutMax=[]  DivideOutMin=[]  DivideOutMax=[]  UdiffTsProdOutMin=[]  UdiffTsProdOutMax=[]  NTsProdOutMin=[]  NTsProdOutMax=[]  UintegralTsProdOutMin=[]  UintegralTsProdOutMax=[]  UngainTsProdOutMin=[]  UngainTsProdOutMax=[]  IntegratorContinuousStateAttributes=''  IntegratorStateMustResolveToSignalObject=off  IntegratorRTWStateStorageClass=Auto  FilterContinuousStateAttributes=''  FilterStateMustResolveToSignalObject=off  FilterRTWStateStorageClass=Auto  ParallelPVariant=InternalParameters  IdealPVariant=Disabled  IVariant=InternalParameters  DVariant=InternalParameters  IntegratorVariant=Discrete  SatVariant=Disabled  AWVariant=Passthrough  PCopyVariant=Disabled  TRVariant=Disabled  FdbkBlocksVariant=Forward  IdealPFdbkVariant=Disabled  SatFdbkVariant=Disabled  DerivativeFilterVariant=ForwardEulerFilter  NVariant=InternalParameters  NCopyVariant=Disabled  FilterICVariant=InternalICsFilter  IntegratorICVariant=InternalICs  ExternalResetVariant=Disabled  TRSumVariant=Passthrough  SumFdbkVariant=Disabled  SumVariant=Sum_PID  TsampFilterVariant=InternalTs  TsampNgainVariant=Passthrough  TsampIntegralVariant=Passthrough  ExternalSaturationOutDataTypeStr=Inherit: Same as second input
  Saturation : Saturate  UpperLimit=Rollrate.intupper  LowerLimit=Rollrate.intlower
  Scope : Scope  NumInputPorts=2
  Sum : Sum  Inputs=|++
  y : Outport
  wires:
  Saturation/1 -> Scope/1, Sum/2
  PID Controller1/1 -> Saturation/1, Scope/2
  Sum/1 -> y/1
  u/1 -> PID Controller2/1, PID Controller1/1
  PID Controller2/1 -> Sum/1

== system CrazyClover_attitude_control_descrete/controller thrust and angular velocity/Attitude rate PID/Yaw rate PID  ==
  u : Inport
  PID Controller : pid_lib/PID Controller  Controller=PID  Form=Parallel  TimeDomain=Discrete-time  UseExternalTs=off  SampleTime=-1  IntegratorMethod=Forward Euler  FilterMethod=Forward Euler  ControllerParametersSource=internal  P=0  I=Yawrate.ki  D=0  UseFilter=on  N=100  TunerSelectOption=Transfer Function Based (PID Tuner App)  InitialConditionSource=internal  InitialConditionForIntegrator=0  InitialConditionForFilter=0  DifferentiatorICPrevScaledInput=0  ExternalReset=none  TrackingMode=off  Kt=1  LimitOutput=off  SatLimitsSource=internal  UpperSaturationLimit=inf  LowerSaturationLimit=-inf  LinearizeAsGain=on  AntiWindupMode=none  Kb=1  POutMin=[]  POutMax=[]  IOutMin=[]  IOutMax=[]  DOutMin=[]  DOutMax=[]  NOutMin=[]  NOutMax=[]  SumOutMin=[]  SumOutMax=[]  SaturationOutMin=[]  SaturationOutMax=[]  PParamMin=[]  PParamMax=[]  IParamMin=[]  IParamMax=[]  DParamMin=[]  DParamMax=[]  NParamMin=[]  NParamMax=[]  KbParamMin=[]  KbParamMax=[]  KtParamMin=[]  KtParamMax=[]  KbOutMin=[]  KbOutMax=[]  KtOutMin=[]  KtOutMax=[]  IntegratorOutMin=[]  IntegratorOutMax=[]  FilterOutMin=[]  FilterOutMax=[]  SumI1OutMin=[]  SumI1OutMax=[]  SumI2OutMin=[]  SumI2OutMax=[]  SumI3OutMin=[]  SumI3OutMax=[]  SumI4OutMin=[]  SumI4OutMax=[]  SumDOutMin=[]  SumDOutMax=[]  DifferentiatorOutMin=[]  DifferentiatorOutMax=[]  FilterDiffOutCoefMin=[]  FilterDiffOutCoefMax=[]  ReciprocalOutMin=[]  ReciprocalOutMax=[]  SumDenOutMin=[]  SumDenOutMax=[]  SumNumOutMin=[]  SumNumOutMax=[]  DivideOutMin=[]  DivideOutMax=[]  UdiffTsProdOutMin=[]  UdiffTsProdOutMax=[]  NTsProdOutMin=[]  NTsProdOutMax=[]  UintegralTsProdOutMin=[]  UintegralTsProdOutMax=[]  UngainTsProdOutMin=[]  UngainTsProdOutMax=[]  IntegratorContinuousStateAttributes=''  IntegratorStateMustResolveToSignalObject=off  IntegratorRTWStateStorageClass=Auto  FilterContinuousStateAttributes=''  FilterStateMustResolveToSignalObject=off  FilterRTWStateStorageClass=Auto  ParallelPVariant=InternalParameters  IdealPVariant=Disabled  IVariant=InternalParameters  DVariant=InternalParameters  IntegratorVariant=Discrete  SatVariant=Disabled  AWVariant=Passthrough  PCopyVariant=Disabled  TRVariant=Disabled  FdbkBlocksVariant=Forward  IdealPFdbkVariant=Disabled  SatFdbkVariant=Disabled  DerivativeFilterVariant=ForwardEulerFilter  NVariant=InternalParameters  NCopyVariant=Disabled  FilterICVariant=InternalICsFilter  IntegratorICVariant=InternalICs  ExternalResetVariant=Disabled  TRSumVariant=Passthrough  SumFdbkVariant=Disabled  SumVariant=Sum_PID  TsampFilterVariant=InternalTs  TsampNgainVariant=Passthrough  TsampIntegralVariant=Passthrough  ExternalSaturationOutDataTypeStr=Inherit: Same as second input
  PID Controller2 : pid_lib/PID Controller  Controller=PID  Form=Parallel  TimeDomain=Discrete-time  UseExternalTs=off  SampleTime=-1  IntegratorMethod=Forward Euler  FilterMethod=Forward Euler  ControllerParametersSource=internal  P=Yawrate.kp  I=0  D=0  UseFilter=on  N=100  TunerSelectOption=Transfer Function Based (PID Tuner App)  InitialConditionSource=internal  InitialConditionForIntegrator=0  InitialConditionForFilter=0  DifferentiatorICPrevScaledInput=0  ExternalReset=none  TrackingMode=off  Kt=1  LimitOutput=off  SatLimitsSource=internal  UpperSaturationLimit=inf  LowerSaturationLimit=-inf  LinearizeAsGain=on  AntiWindupMode=none  Kb=1  POutMin=[]  POutMax=[]  IOutMin=[]  IOutMax=[]  DOutMin=[]  DOutMax=[]  NOutMin=[]  NOutMax=[]  SumOutMin=[]  SumOutMax=[]  SaturationOutMin=[]  SaturationOutMax=[]  PParamMin=[]  PParamMax=[]  IParamMin=[]  IParamMax=[]  DParamMin=[]  DParamMax=[]  NParamMin=[]  NParamMax=[]  KbParamMin=[]  KbParamMax=[]  KtParamMin=[]  KtParamMax=[]  KbOutMin=[]  KbOutMax=[]  KtOutMin=[]  KtOutMax=[]  IntegratorOutMin=[]  IntegratorOutMax=[]  FilterOutMin=[]  FilterOutMax=[]  SumI1OutMin=[]  SumI1OutMax=[]  SumI2OutMin=[]  SumI2OutMax=[]  SumI3OutMin=[]  SumI3OutMax=[]  SumI4OutMin=[]  SumI4OutMax=[]  SumDOutMin=[]  SumDOutMax=[]  DifferentiatorOutMin=[]  DifferentiatorOutMax=[]  FilterDiffOutCoefMin=[]  FilterDiffOutCoefMax=[]  ReciprocalOutMin=[]  ReciprocalOutMax=[]  SumDenOutMin=[]  SumDenOutMax=[]  SumNumOutMin=[]  SumNumOutMax=[]  DivideOutMin=[]  DivideOutMax=[]  UdiffTsProdOutMin=[]  UdiffTsProdOutMax=[]  NTsProdOutMin=[]  NTsProdOutMax=[]  UintegralTsProdOutMin=[]  UintegralTsProdOutMax=[]  UngainTsProdOutMin=[]  UngainTsProdOutMax=[]  IntegratorContinuousStateAttributes=''  IntegratorStateMustResolveToSignalObject=off  IntegratorRTWStateStorageClass=Auto  FilterContinuousStateAttributes=''  FilterStateMustResolveToSignalObject=off  FilterRTWStateStorageClass=Auto  ParallelPVariant=InternalParameters  IdealPVariant=Disabled  IVariant=InternalParameters  DVariant=InternalParameters  IntegratorVariant=Discrete  SatVariant=Disabled  AWVariant=Passthrough  PCopyVariant=Disabled  TRVariant=Disabled  FdbkBlocksVariant=Forward  IdealPFdbkVariant=Disabled  SatFdbkVariant=Disabled  DerivativeFilterVariant=ForwardEulerFilter  NVariant=InternalParameters  NCopyVariant=Disabled  FilterICVariant=InternalICsFilter  IntegratorICVariant=InternalICs  ExternalResetVariant=Disabled  TRSumVariant=Passthrough  SumFdbkVariant=Disabled  SumVariant=Sum_PID  TsampFilterVariant=InternalTs  TsampNgainVariant=Passthrough  TsampIntegralVariant=Passthrough  ExternalSaturationOutDataTypeStr=Inherit: Same as second input
  Saturation : Saturate  UpperLimit=Yawrate.intupper  LowerLimit=Yawrate.intlower
  Scope : Scope  NumInputPorts=2
  Sum : Sum  Inputs=|++
  y : Outport
  wires:
  PID Controller2/1 -> Sum/1
  u/1 -> PID Controller/1, PID Controller2/1
  Sum/1 -> y/1
  PID Controller/1 -> Scope/2, Saturation/1
  Saturation/1 -> Sum/2, Scope/1

== system CrazyClover_attitude_control_descrete/controller thrust and angular velocity/Attitude rate PID/pitch rate PID ==
  u : Inport
  PID Controller1 : pid_lib/PID Controller  Controller=PID  Form=Parallel  TimeDomain=Discrete-time  UseExternalTs=off  SampleTime=-1  IntegratorMethod=Forward Euler  FilterMethod=Forward Euler  ControllerParametersSource=internal  P=0  I=Pitchrate.ki  D=0  UseFilter=on  N=100  TunerSelectOption=Transfer Function Based (PID Tuner App)  InitialConditionSource=internal  InitialConditionForIntegrator=0  InitialConditionForFilter=0  DifferentiatorICPrevScaledInput=0  ExternalReset=none  TrackingMode=off  Kt=1  LimitOutput=off  SatLimitsSource=internal  UpperSaturationLimit=inf  LowerSaturationLimit=-inf  LinearizeAsGain=on  AntiWindupMode=none  Kb=1  POutMin=[]  POutMax=[]  IOutMin=[]  IOutMax=[]  DOutMin=[]  DOutMax=[]  NOutMin=[]  NOutMax=[]  SumOutMin=[]  SumOutMax=[]  SaturationOutMin=[]  SaturationOutMax=[]  PParamMin=[]  PParamMax=[]  IParamMin=[]  IParamMax=[]  DParamMin=[]  DParamMax=[]  NParamMin=[]  NParamMax=[]  KbParamMin=[]  KbParamMax=[]  KtParamMin=[]  KtParamMax=[]  KbOutMin=[]  KbOutMax=[]  KtOutMin=[]  KtOutMax=[]  IntegratorOutMin=[]  IntegratorOutMax=[]  FilterOutMin=[]  FilterOutMax=[]  SumI1OutMin=[]  SumI1OutMax=[]  SumI2OutMin=[]  SumI2OutMax=[]  SumI3OutMin=[]  SumI3OutMax=[]  SumI4OutMin=[]  SumI4OutMax=[]  SumDOutMin=[]  SumDOutMax=[]  DifferentiatorOutMin=[]  DifferentiatorOutMax=[]  FilterDiffOutCoefMin=[]  FilterDiffOutCoefMax=[]  ReciprocalOutMin=[]  ReciprocalOutMax=[]  SumDenOutMin=[]  SumDenOutMax=[]  SumNumOutMin=[]  SumNumOutMax=[]  DivideOutMin=[]  DivideOutMax=[]  UdiffTsProdOutMin=[]  UdiffTsProdOutMax=[]  NTsProdOutMin=[]  NTsProdOutMax=[]  UintegralTsProdOutMin=[]  UintegralTsProdOutMax=[]  UngainTsProdOutMin=[]  UngainTsProdOutMax=[]  IntegratorContinuousStateAttributes=''  IntegratorStateMustResolveToSignalObject=off  IntegratorRTWStateStorageClass=Auto  FilterContinuousStateAttributes=''  FilterStateMustResolveToSignalObject=off  FilterRTWStateStorageClass=Auto  ParallelPVariant=InternalParameters  IdealPVariant=Disabled  IVariant=InternalParameters  DVariant=InternalParameters  IntegratorVariant=Discrete  SatVariant=Disabled  AWVariant=Passthrough  PCopyVariant=Disabled  TRVariant=Disabled  FdbkBlocksVariant=Forward  IdealPFdbkVariant=Disabled  SatFdbkVariant=Disabled  DerivativeFilterVariant=ForwardEulerFilter  NVariant=InternalParameters  NCopyVariant=Disabled  FilterICVariant=InternalICsFilter  IntegratorICVariant=InternalICs  ExternalResetVariant=Disabled  TRSumVariant=Passthrough  SumFdbkVariant=Disabled  SumVariant=Sum_PID  TsampFilterVariant=InternalTs  TsampNgainVariant=Passthrough  TsampIntegralVariant=Passthrough  ExternalSaturationOutDataTypeStr=Inherit: Same as second input
  PID Controller2 : pid_lib/PID Controller  Controller=PID  Form=Parallel  TimeDomain=Discrete-time  UseExternalTs=off  SampleTime=-1  IntegratorMethod=Forward Euler  FilterMethod=Forward Euler  ControllerParametersSource=internal  P=Pitchrate.kp  I=0  D=0  UseFilter=on  N=100  TunerSelectOption=Transfer Function Based (PID Tuner App)  InitialConditionSource=internal  InitialConditionForIntegrator=0  InitialConditionForFilter=0  DifferentiatorICPrevScaledInput=0  ExternalReset=none  TrackingMode=off  Kt=1  LimitOutput=off  SatLimitsSource=internal  UpperSaturationLimit=inf  LowerSaturationLimit=-inf  LinearizeAsGain=on  AntiWindupMode=none  Kb=1  POutMin=[]  POutMax=[]  IOutMin=[]  IOutMax=[]  DOutMin=[]  DOutMax=[]  NOutMin=[]  NOutMax=[]  SumOutMin=[]  SumOutMax=[]  SaturationOutMin=[]  SaturationOutMax=[]  PParamMin=[]  PParamMax=[]  IParamMin=[]  IParamMax=[]  DParamMin=[]  DParamMax=[]  NParamMin=[]  NParamMax=[]  KbParamMin=[]  KbParamMax=[]  KtParamMin=[]  KtParamMax=[]  KbOutMin=[]  KbOutMax=[]  KtOutMin=[]  KtOutMax=[]  IntegratorOutMin=[]  IntegratorOutMax=[]  FilterOutMin=[]  FilterOutMax=[]  SumI1OutMin=[]  SumI1OutMax=[]  SumI2OutMin=[]  SumI2OutMax=[]  SumI3OutMin=[]  SumI3OutMax=[]  SumI4OutMin=[]  SumI4OutMax=[]  SumDOutMin=[]  SumDOutMax=[]  DifferentiatorOutMin=[]  DifferentiatorOutMax=[]  FilterDiffOutCoefMin=[]  FilterDiffOutCoefMax=[]  ReciprocalOutMin=[]  ReciprocalOutMax=[]  SumDenOutMin=[]  SumDenOutMax=[]  SumNumOutMin=[]  SumNumOutMax=[]  DivideOutMin=[]  DivideOutMax=[]  UdiffTsProdOutMin=[]  UdiffTsProdOutMax=[]  NTsProdOutMin=[]  NTsProdOutMax=[]  UintegralTsProdOutMin=[]  UintegralTsProdOutMax=[]  UngainTsProdOutMin=[]  UngainTsProdOutMax=[]  IntegratorContinuousStateAttributes=''  IntegratorStateMustResolveToSignalObject=off  IntegratorRTWStateStorageClass=Auto  FilterContinuousStateAttributes=''  FilterStateMustResolveToSignalObject=off  FilterRTWStateStorageClass=Auto  ParallelPVariant=InternalParameters  IdealPVariant=Disabled  IVariant=InternalParameters  DVariant=InternalParameters  IntegratorVariant=Discrete  SatVariant=Disabled  AWVariant=Passthrough  PCopyVariant=Disabled  TRVariant=Disabled  FdbkBlocksVariant=Forward  IdealPFdbkVariant=Disabled  SatFdbkVariant=Disabled  DerivativeFilterVariant=ForwardEulerFilter  NVariant=InternalParameters  NCopyVariant=Disabled  FilterICVariant=InternalICsFilter  IntegratorICVariant=InternalICs  ExternalResetVariant=Disabled  TRSumVariant=Passthrough  SumFdbkVariant=Disabled  SumVariant=Sum_PID  TsampFilterVariant=InternalTs  TsampNgainVariant=Passthrough  TsampIntegralVariant=Passthrough  ExternalSaturationOutDataTypeStr=Inherit: Same as second input
  Saturation : Saturate  UpperLimit=Pitchrate.intupper  LowerLimit=Pitchrate.intlower
  Scope : Scope  NumInputPorts=2
  Sum : Sum  Inputs=|++
  y : Outport
  wires:
  PID Controller2/1 -> Sum/1
  u/1 -> PID Controller1/1, PID Controller2/1
  Sum/1 -> y/1
  PID Controller1/1 -> Scope/2, Saturation/1
  Saturation/1 -> Sum/2, Scope/1
